simulink model "Baseball_Sim2"  (R2025a)
settings: Solver=ode45  StartTime=0.0  StopTime=10.0  MaxStep=0.0001  RelTol=1e-5  AbsTol=1e-8
undefined symbols (not defined in the file): initialVelocity, releaseHeight, spinAngle, spinRate
libraries: simulink x1
settings Model: Creator=aahilkeshwani  LastModifiedBy=aahilkeshwani

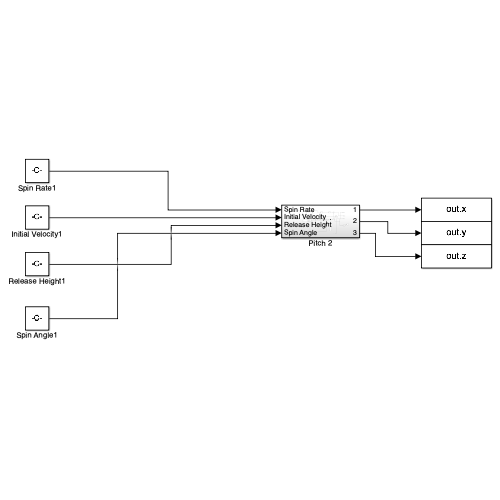
[thumbnail: Simulink's stored preview of the top-level diagram]
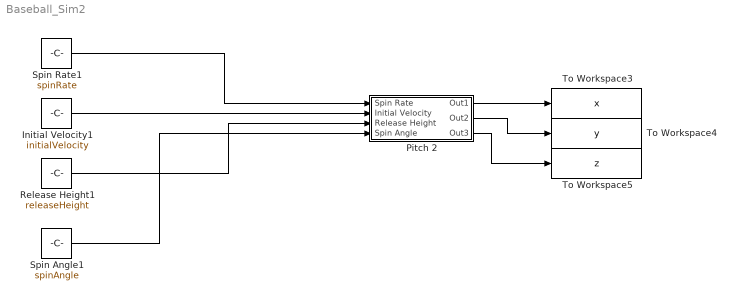
== system Baseball_Sim2 ==
  Initial Velocity1 : Constant  Value=initialVelocity
  Pitch 2 : Subsystem
  Release Height1 : Constant  Value=releaseHeight
  Spin Angle1 : Constant  Value=spinAngle
  Spin Rate1 : Constant  Value=spinRate
  To Workspace3 : ToWorkspace  VariableName=x  SampleTime=-1
  To Workspace4 : ToWorkspace  VariableName=y  SampleTime=-1
  To Workspace5 : ToWorkspace  VariableName=z  SampleTime=-1
  wires:
  Spin Angle1/1 -> Pitch 2/4(Spin Angle)
  Release Height1/1 -> Pitch 2/3(Release Height)
  Initial Velocity1/1 -> Pitch 2/2(Initial Velocity)
  Spin Rate1/1 -> Pitch 2/1(Spin Rate)
  Pitch 2/1(Out1) -> To Workspace3/1
  Pitch 2/3(Out3) -> To Workspace5/1
  Pitch 2/2(Out2) -> To Workspace4/1

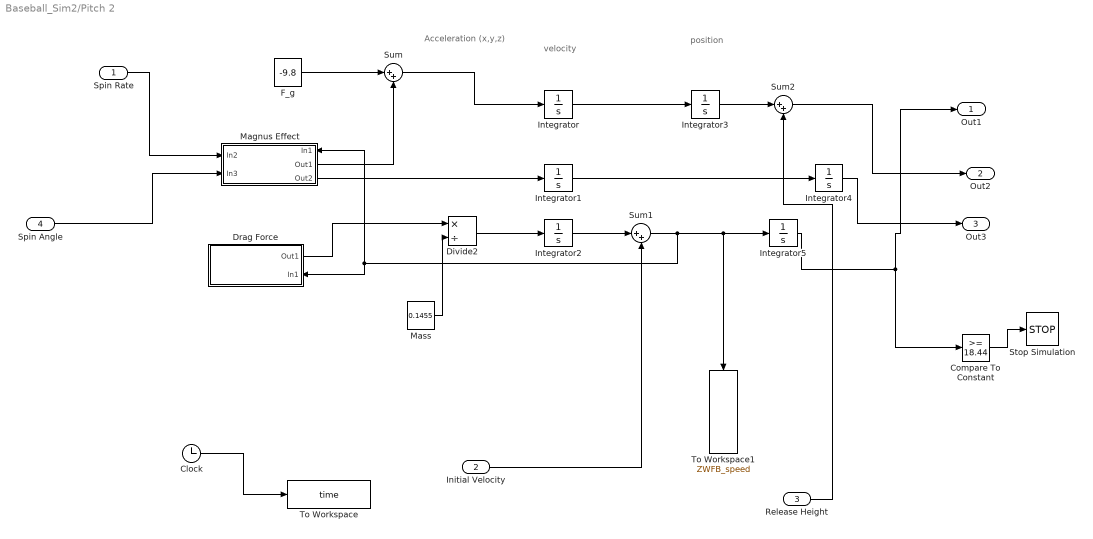
== system Baseball_Sim2/Pitch 2 ==
  note: velocity
  note: Acceleration (x,y,z)
  note: position
  Spin Rate : Inport
  Initial Velocity : Inport  Port=2
  Release Height : Inport  Port=3
  Spin Angle : Inport  Port=4
  Clock : Clock
  Compare To Constant : simulink/Logic and Bit Operations/Compare To Constant  relop=>=  const=18.44  OutDataTypeStr=boolean
  Divide2 : Product  Inputs=*/
  Drag Force : Subsystem
      settings: PortSchema="{\"entries\":[{\"content\":{\"sides\":[{\"content\":{\"connectorIds\":[\"Out1\",\"In1\"]},\"type\":\"ConnectorPlacement.EquallySpacedRectSide\",\"uuid\":\"216831b0-24e3-4aea-a273-c3106f64cd54\"},{\"content\":{\"side\":\"RIGHT\"},\"type\":\"ConnectorPlacement.EquallySpacedRectSide\",\"uuid\":\"10ad226f-4bf7-4a19-a8e5-d24de9a5a893\"},{\"content\":{\"side\":\"TOP\"},\"type\":\"ConnectorPlacement.EquallySpacedRectSide\",\"uuid\":\"0a6683d0-3335-45e1-997a-6db41e3e08c7\"}]},\"type\":\"ConnectorPlacement.EquallySpacedConnector\",\"uuid\":\"93f05356-acc4-47b4-a72e-aa46317d3351\"}],\"packageUris\":[\"http://schema.mathworks.com/mf0/Connector/R2020b\"],\"version\":\"1.0\"}"
  F_g : Constant  Value=-9.8
  Integrator{,1..5} (6 alike) : Integrator
  Magnus Effect : Subsystem
      settings: PortSchema="{\"entries\":[{\"content\":{\"sides\":[{\"content\":{\"connectorIds\":[\"In1\",\"Out1\",\"Out2\"]},\"type\":\"ConnectorPlacement.EquallySpacedRectSide\",\"uuid\":\"98f08cfc-7b60-4007-860c-95789bd91ec7\"},{\"content\":{\"connectorIds\":[\"In2\",\"In3\"],\"side\":\"RIGHT\"},\"type\":\"ConnectorPlacement.EquallySpacedRectSide\",\"uuid\":\"bf6b90cb-5bdf-4e75-8697-2db2bc3d2708\"},{\"content\":{\"side\":\"TOP\"},\"type\":\"ConnectorPlacement.EquallySpacedRectSide\",\"uuid\":\"68cdd1d5-0d03-40c0-8112-70f031e7c219\"},{\"content\":{\"side\":\"BOTTOM\"},\"type\":\"ConnectorPlacement.EquallySpacedRectSide\",\"uuid\":\"a393b2e2-478f-45bd-8f12-982876140266\"}]},\"type\":\"ConnectorPlacement.EquallySpacedConnector\",\"uuid\":\"dbb95a60-0430-4631-9ffe-3248640cd1a4\"}],\"packageUris\":[\"http://schema.mathworks.com/mf0/Connector/R2020b\"],\"version\":\"1.0\"}"
  Mass : Constant  Value=0.1455
  Stop Simulation : Stop
  Sum : Sum  Inputs=|++
  Sum1 : Sum  Inputs=|++
  Sum2 : Sum  Inputs=|++
  To Workspace : ToWorkspace  VariableName=time  SampleTime=-1
  To Workspace1 : ToWorkspace  VariableName=ZWFB_speed  SaveFormat=Timeseries  SampleTime=-1
  Out1 : Outport
  Out2 : Outport  Port=2
  Out3 : Outport  Port=3
  wires:
  Sum1/1 -> Drag Force/1(In1), Magnus Effect/1(In1), Integrator5/1, To Workspace1/1
  F_g/1 -> Sum/1
  Drag Force/1(Out1) -> Divide2/1
  Integrator2/1 -> Sum1/1
  Integrator3/1 -> Sum2/1
  Integrator1/1 -> Integrator4/1
  Divide2/1 -> Integrator2/1
  Magnus Effect/2(Out2) -> Integrator1/1
  Spin Angle/1 -> Magnus Effect/3(In3)
  Initial Velocity/1 -> Sum1/2
  Sum/1 -> Integrator/1
  Integrator/1 -> Integrator3/1
  Mass/1 -> Divide2/2
  Release Height/1 -> Sum2/2
  Magnus Effect/1(Out1) -> Sum/2
  Spin Rate/1 -> Magnus Effect/2(In2)
  Integrator5/1 -> Out1/1, Compare To Constant/1
  Sum2/1 -> Out2/1
  Integrator4/1 -> Out3/1
  Compare To Constant/1 -> Stop Simulation/1
  Clock/1 -> To Workspace/1

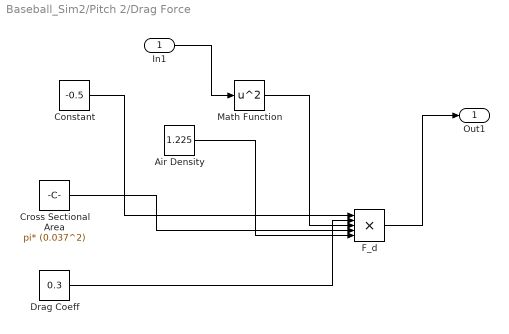
== system Baseball_Sim2/Pitch 2/Drag Force ==
  In1 : Inport
  Air Density : Constant  Value=1.225
  Constant : Constant  Value=-0.5
  Cross Sectional Area : Constant  Value=pi* (0.037^2)
  Drag Coeff : Constant  Value=0.3
  F_d : Product  Inputs=5
  Math Function : Math  Operator=square
  Out1 : Outport
  wires:
  In1/1 -> Math Function/1
  Cross Sectional Area/1 -> F_d/4
  Constant/1 -> F_d/1
  Drag Coeff/1 -> F_d/2
  Air Density/1 -> F_d/5
  Math Function/1 -> F_d/3
  F_d/1 -> Out1/1

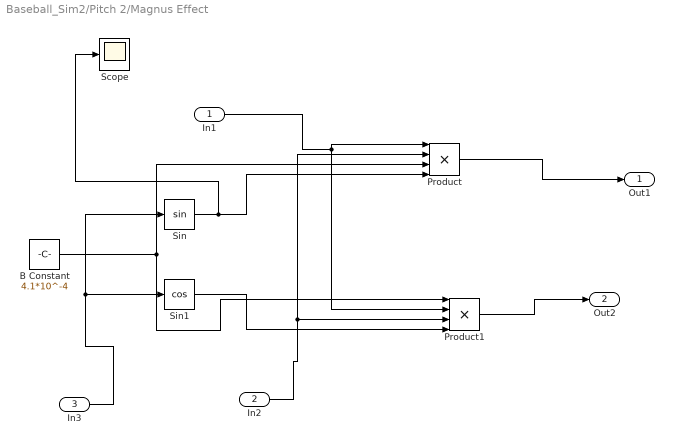
== system Baseball_Sim2/Pitch 2/Magnus Effect ==
  In1 : Inport
  In2 : Inport  Port=2
  In3 : Inport  Port=3
  B Constant : Constant  Value=4.1*10^-4
  Product : Product  Inputs=4
  Product1 : Product  Inputs=4
  Scope : Scope
      settings: ActiveDisplayYMinimum=0.9  ActiveDisplayYMaximum=1.1
  Sin : Trigonometry
  Sin1 : Trigonometry  Operator=cos
  Out1 : Outport
  Out2 : Outport  Port=2
  wires:
  In1/1 -> Product1/2, Product/1
  In3/1 -> Sin/1, Sin1/1
  Sin/1 -> Scope/1, Product/4
  Sin1/1 -> Product1/4
  B Constant/1 -> Product1/1, Product/3
  In2/1 -> Product1/3, Product/2
  Product/1 -> Out1/1
  Product1/1 -> Out2/1
